simulink model "Testing"  (R2024a)
settings: Solver=VariableStepAuto  StartTime=0.0  StopTime=10.0  RelTol=1e-3
libraries: opcualib x1
settings Model: Creator=guilh  LastModifiedBy=guilh

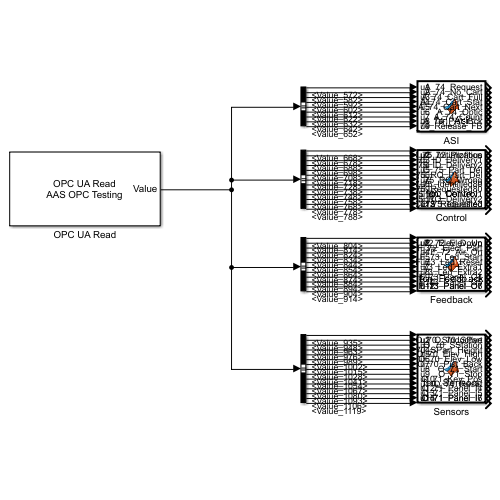
[thumbnail: Simulink's stored preview of the top-level diagram]
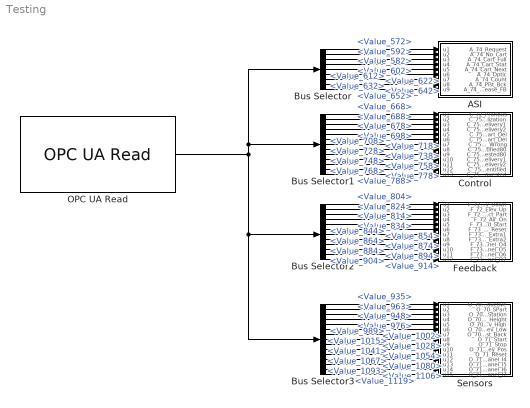
== system Testing ==
  ASI : MATLAB Function  TreatAsAtomicUnit=on
  Bus Selector : BusSelector  OutputSignals=Value_572,Value_582,Value_592,Value_602,Value_612,Value_622,Value_632,Value_642,Value_652
  Bus Selector1 : BusSelector  OutputSignals=Value_668,Value_678,Value_688,Value_698,Value_708,Value_718,Value_728,Value_738,Value_748,Value_758,Value_768,Value_778,Value_788
  Bus Selector2 : BusSelector  OutputSignals=Value_804,Value_814,Value_824,Value_834,Value_844,Value_854,Value_864,Value_874,Value_884,Value_894,Value_904,Value_914
  Bus Selector3 : BusSelector  OutputSignals=Value_935,Value_948,Value_963,Value_976,Value_989,Value_1002,Value_1015,Value_1028,Value_1041,Value_1054,Value_1067,Value_1080,Value_1093,Value_1106,Value_1119
  Control : MATLAB Function  TreatAsAtomicUnit=on
  Feedback : MATLAB Function  TreatAsAtomicUnit=on
  OPC UA Read : opcualib/OPC UA Read  SelectedServer=AAS OPC Testing  ServerList=AAS OPC Testing  NodeList={ '1', 'Value', '6', '572', '1'; '2', 'Value', '6', '582', '1'; '3', 'Value', '6', '592', '1'; '4', 'Value', '6', '602', '1'; '5', 'Value', '6', '612', '1'; '6', 'Value', '6', '622', '1'; '7', 'Value', '6', '632', '1'; '8', 'Value', '6', '642', '1'; '9', 'Value', '6', '652', '1'; '10', 'Value', '6', '668', '1'; '11', 'Value', '6', '678', '1'; '12', 'Value', '6', '688', '1'; '13', 'Value', '6', '698', '1'; '14', 'Value', '6', '708', '1'; '15', 'Value', '6', '718', '1'; '16', 'Value', '6', '728', '1'; '17', 'Value', '6', '738', '1'; '18', 'Value', '6', '748', '1'; '19', 'Value', '6', '758', '1'; '20', 'Value', '6', '768', '1'; '21', 'Value', '6', '778', '1'; '22', 'Value', '6', '788', '1'; '23', 'Value', '6', '804', '1'; '24', 'Value', '6', '814', '1'; '25', 'Value', '6', '824', '1'; '26', 'Value', '6', '834', '1'; '27', 'Value', '6', '844', '1'; '28', 'Value', '6', '854', '1'; '29', 'Value', '6', '864', '1'; '30', 'Value', '6', '874', '1'; '31', 'Value', '6', '884', '1'; '32', 'Value', '6', '894', '1'; '33', 'Value', '6', '904', '1'; '34', 'Value', '6', '914', '1'; '35', 'Value', '6', '935', '1'; '36', 'Value', '6', '948', '1'; '37', 'Value', '6', '963', '1'; '38', 'Value', '6', '976', '1'; '39', 'Value', '6', '989', '1'; '40', 'Value', '6', '1002', '1'; '41', 'Value', '6', '1015', '1'; '42', 'Value', '6', '1028', '1'; '43', 'Value', '6', '1041', '1'; '44', 'Value', '6', '1054', '1'; '45', 'Value', '6', '1067', '1'; '46', 'Value', '6', '1080', '1'; '47', 'Value', '6', '1093', '1'; '48', 'Value', '6', '1106', '1'; '49', 'Value', '6', '1119', '1' }  ShowQualityPort=off  ShowTimestampPort=off  ShowTimestampPortAs=Seconds since start  SampleTime=-1
  Sensors : MATLAB Function  TreatAsAtomicUnit=on
  wires:
  OPC UA Read/1 -> Bus Selector3/1, Bus Selector2/1, Bus Selector1/1, Bus Selector/1
  Bus Selector/1 -> ASI/1(u1)  "<Value_572>"
  Bus Selector/2 -> ASI/2(u2)  "<Value_582>"
  Bus Selector/3 -> ASI/3(u3)  "<Value_592>"
  Bus Selector/4 -> ASI/4(u4)  "<Value_602>"
  Bus Selector/5 -> ASI/5(u5)  "<Value_612>"
  Bus Selector/6 -> ASI/6(u6)  "<Value_622>"
  Bus Selector/7 -> ASI/7(u7)  "<Value_632>"
  Bus Selector/8 -> ASI/8(u8)  "<Value_642>"
  Bus Selector/9 -> ASI/9(u9)  "<Value_652>"
  Bus Selector1/1 -> Control/1(u1)  "<Value_668>"
  Bus Selector1/2 -> Control/2(u2)  "<Value_678>"
  Bus Selector1/3 -> Control/3(u3)  "<Value_688>"
  Bus Selector1/4 -> Control/4(u4)  "<Value_698>"
  Bus Selector1/5 -> Control/5(u5)  "<Value_708>"
  Bus Selector1/6 -> Control/6(u6)  "<Value_718>"
  Bus Selector1/7 -> Control/7(u7)  "<Value_728>"
  Bus Selector1/8 -> Control/8(u8)  "<Value_738>"
  Bus Selector1/9 -> Control/9(u9)  "<Value_748>"
  Bus Selector1/10 -> Control/10(u10)  "<Value_758>"
  Bus Selector1/11 -> Control/11(u11)  "<Value_768>"
  Bus Selector1/12 -> Control/12(u12)  "<Value_778>"
  Bus Selector1/13 -> Control/13(u13)  "<Value_788>"
  Bus Selector2/1 -> Feedback/1(u1)  "<Value_804>"
  Bus Selector2/2 -> Feedback/2(u2)  "<Value_814>"
  Bus Selector2/3 -> Feedback/3(u3)  "<Value_824>"
  Bus Selector2/4 -> Feedback/4(u4)  "<Value_834>"
  Bus Selector2/5 -> Feedback/5(u5)  "<Value_844>"
  Bus Selector2/6 -> Feedback/6(u6)  "<Value_854>"
  Bus Selector2/7 -> Feedback/7(u7)  "<Value_864>"
  Bus Selector2/8 -> Feedback/8(u8)  "<Value_874>"
  Bus Selector2/9 -> Feedback/9(u9)  "<Value_884>"
  Bus Selector2/10 -> Feedback/10(u10)  "<Value_894>"
  Bus Selector2/11 -> Feedback/11(u11)  "<Value_904>"
  Bus Selector2/12 -> Feedback/12(u12)  "<Value_914>"
  Bus Selector3/1 -> Sensors/1(u1)  "<Value_935>"
  Bus Selector3/2 -> Sensors/2(u2)  "<Value_948>"
  Bus Selector3/3 -> Sensors/3(u3)  "<Value_963>"
  Bus Selector3/4 -> Sensors/4(u4)  "<Value_976>"
  Bus Selector3/5 -> Sensors/5(u5)  "<Value_989>"
  Bus Selector3/6 -> Sensors/6(u6)  "<Value_1002>"
  Bus Selector3/7 -> Sensors/7(u7)  "<Value_1015>"
  Bus Selector3/8 -> Sensors/8(u8)  "<Value_1028>"
  Bus Selector3/9 -> Sensors/9(u9)  "<Value_1041>"
  Bus Selector3/10 -> Sensors/10(u10)  "<Value_1054>"
  Bus Selector3/11 -> Sensors/11(u11)  "<Value_1067>"
  Bus Selector3/12 -> Sensors/12(u12)  "<Value_1080>"
  Bus Selector3/13 -> Sensors/13(u13)  "<Value_1093>"
  Bus Selector3/14 -> Sensors/14(u14)  "<Value_1106>"
  Bus Selector3/15 -> Sensors/15(u15)  "<Value_1119>"

== matlab function Testing/Sensors ==
  data: u1 input; O_70_SInductive output; u2 input; u3 input; u4 input; u5 input; u6 input; u7 input; u8 input; u9 input; u10 input; u11 input; u12 input; u13 input; u14 input; u15 input; O_70_SPart output; O_70_SStation output; O_70_SPart_Height output; O_70_Elev_High output; O_70_Elev_Low output; O_70_Pist_Back output; O_71_Start output; O_71_Stop output; O_71_Key_Pos output; O_71_Reset output; O_71_Panel_I4 output; O_71_Panel_I5 output; O_71_Panel_I6 output; O_71_Panel_I7 output
function [O_70_SInductive, O_70_SPart, O_70_SStation, O_70_SPart_Height, ...
          O_70_Elev_High, O_70_Elev_Low, O_70_Pist_Back, O_71_Start, ...
          O_71_Stop, O_71_Key_Pos, O_71_Reset, O_71_Panel_I4, O_71_Panel_I5, ...
          O_71_Panel_I6, O_71_Panel_I7] = ...
          fcn_Sensors(u1, u2, u3, u4, u5, u6, u7, u8, u9, u10, ...
          u11, u12, u13, u14, u15)

O_70_SInductive = u1;
O_70_SPart = u2;
O_70_SStation = u3;
O_70_SPart_Height = u4;
O_70_Elev_High = u5;
O_70_Elev_Low = u6;
O_70_Pist_Back = u7;
O_71_Start = u8;
O_71_Stop = u9;
O_71_Key_Pos = u10;
O_71_Reset = u11;
O_71_Panel_I4 = u12;
O_71_Panel_I5 = u13;
O_71_Panel_I6 = u14;
O_71_Panel_I7 = u15;

== matlab function Testing/Control ==
  data: u1 input; C_72_Profibus output; u2 input; u3 input; u4 input; u5 input; u6 input; u7 input; u8 input; u9 input; u10 input; u11 input; u12 input; u13 input; C_75_Initialization output; C_75_ID_Delivery1 output; C_75_ID_Delivery2 output; C_75_Part_Del output; C_75_RQ_Part_Del output; C_75_RQ_Wrong output; C_75_Identified80 output; C_75_Requested80 output; C_75_RQ_Delivery1 output; C_75_RQ_Delivery2 output; C_75_Identified output; C_75_Requested output
function [C_72_Profibus, C_75_Initialization, C_75_ID_Delivery1, C_75_ID_Delivery2, ...
          C_75_Part_Del, C_75_RQ_Part_Del, C_75_RQ_Wrong, C_75_Identified80, ...
          C_75_Requested80, C_75_RQ_Delivery1, C_75_RQ_Delivery2, C_75_Identified, ...
          C_75_Requested] = fcn_Control(u1, u2, u3, u4, u5, u6, u7, u8, u9, u10, u11, u12, u13)

C_72_Profibus = u1;
C_75_Initialization = u2;
C_75_ID_Delivery1 = u3;
C_75_ID_Delivery2 = u4;
C_75_Part_Del = u5;
C_75_RQ_Part_Del = u6;
C_75_RQ_Wrong = u7;
C_75_Identified80 = u8;
C_75_Requested80 = u9;
C_75_RQ_Delivery1 = u10;
C_75_RQ_Delivery2 = u11;
C_75_Identified = u12;
C_75_Requested = u13;

== matlab function Testing/ASI ==
  data: u1 input; A_74_Request output; u2 input; u3 input; u4 input; u5 input; u6 input; u7 input; u8 input; u9 input; A_74_No_Cart output; A_74_Cart_Full output; A_74_Cart_Stat output; A_74_Cart_Next output; A_74_Optic output; A_74_Count output; A_74_Pist_Bck output; A_74_Release_FB output
function [A_74_Request, A_74_No_Cart, A_74_Cart_Full, A_74_Cart_Stat, ...
          A_74_Cart_Next, A_74_Optic, A_74_Count, A_74_Pist_Bck, ...
          A_74_Release_FB] = fcn_Asi(u1, u2, u3, u4, u5, u6, u7, u8, u9)

A_74_Request = u1;
A_74_No_Cart = u2;
A_74_Cart_Full = u3;
A_74_Cart_Stat = u4;
A_74_Cart_Next = u5;
A_74_Optic = u6;
A_74_Count = u7;
A_74_Pist_Bck = u8;
A_74_Release_FB = u9;

== matlab function Testing/Feedback ==
  data: u1 input; F_72_Elev_Down output; u2 input; u3 input; u4 input; u5 input; u6 input; u7 input; u8 input; u9 input; u10 input; u11 input; u12 input; F_72_Elev_Up output; F_72_Eject_Part output; F_72_Air_On output; F_73_Led_Start output; F_73_Led_Reset output; F_73_Led_Extra1 output; F_73_Led_Extra2 output; F_73_Panel_O4 output; F_73_Panel_O5 output; F_73_Panel_O6 output; F_73_Panel_O7 output
function [F_72_Elev_Down, F_72_Elev_Up, F_72_Eject_Part, F_72_Air_On, ...
          F_73_Led_Start, F_73_Led_Reset, F_73_Led_Extra1, F_73_Led_Extra2, ...
          F_73_Panel_O4, F_73_Panel_O5, F_73_Panel_O6, F_73_Panel_O7] = ...
          fcn_Feedback(u1, u2, u3, u4, u5, u6, u7, u8, u9, u10, u11, u12)

F_72_Elev_Down = u1;
F_72_Elev_Up = u2;
F_72_Eject_Part = u3;
F_72_Air_On = u4;
F_73_Led_Start = u5;
F_73_Led_Reset = u6;
F_73_Led_Extra1 = u7;
F_73_Led_Extra2 = u8;
F_73_Panel_O4 = u9;
F_73_Panel_O5 = u10;
F_73_Panel_O6 = u11;
F_73_Panel_O7 = u12;
